simulink model "One_level_boost_igbt_shortcircuit"  (R2022a)
settings: Solver=VariableStepAuto  StartTime=0.0  StopTime=10  MaxStep=10e-6  RelTol=1e-3
libraries: spsSeriesRLCBranchLib x3, spsCurrentMeasurementLib x2, spsDiodeLib x1, spsIdealSwitchLib x1, spsDCVoltageSourceLib x1, spsVoltageMeasurementLib x1, spspowerguiLib x1
settings Model: Creator=Andris  LastModifiedBy=Andris

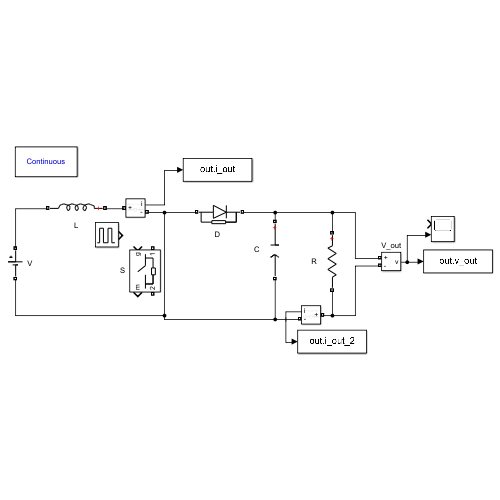
[thumbnail: Simulink's stored preview of the top-level diagram]
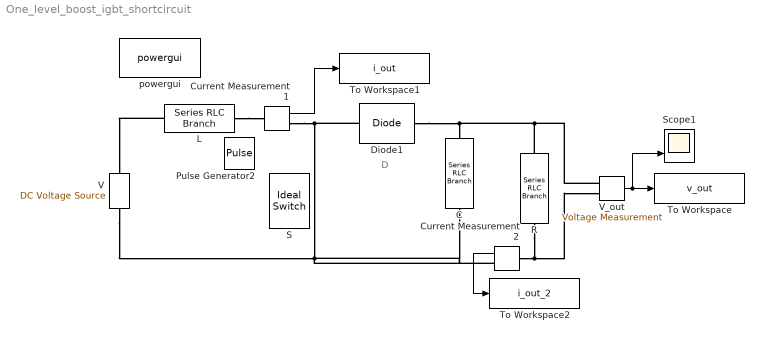
== system One_level_boost_igbt_shortcircuit ==
  note: D
  C : spsSeriesRLCBranchLib/Series RLC Branch  LConnTagsString=__new0  RConnTagsString=__new0  BranchType=C  Resistance=1  Inductance=1e-3  SetiL0=off  InitialCurrent=0  Capacitance=220e-6  Setx0=off  InitialVoltage=Vop1  Measurements=None
  Current Measurement1 : spsCurrentMeasurementLib/Current Measurement  PhasorSimulation=off  OutputType=Complex  PSBequivalent=0
  Current Measurement2 : spsCurrentMeasurementLib/Current Measurement  PhasorSimulation=off  OutputType=Complex  PSBequivalent=0
  Diode1 : spsDiodeLib/Diode  Ron=0  Lon=0  Vf=0  IC=0  UseSnubber=off  Rs=100000  Cs=inf  Measurements=off
  L : spsSeriesRLCBranchLib/Series RLC Branch  LConnTagsString=__new0  RConnTagsString=__new0  BranchType=L  Resistance=1  Inductance=50e-6  SetiL0=off  InitialCurrent=0  Capacitance=1e-6  Setx0=off  InitialVoltage=0  Measurements=None
  Pulse Generator2 : DiscretePulseGenerator  PulseType=Time based  Period=1/48000  PulseWidth=50
  R : spsSeriesRLCBranchLib/Series RLC Branch  LConnTagsString=__new0  RConnTagsString=__new0  BranchType=R  Resistance=12.5  Inductance=1e-3  SetiL0=off  InitialCurrent=0  Capacitance=1e-6  Setx0=off  InitialVoltage=0  Measurements=None
  S : spsIdealSwitchLib/Ideal Switch  Ron=0.001  Lon=0  IC=0  Rs=1e5  Cs=inf  Measurements=on
  Scope1 : Scope  NumInputPorts=2
  To Workspace : ToWorkspace  VariableName=v_out  SampleTime=0.0005
      settings: MaxDataPoints=18000  Save2DSignal=2-D array (concatenate along first dimension)
  To Workspace1 : ToWorkspace  VariableName=i_out  SampleTime=0.0005
      settings: MaxDataPoints=18000  Save2DSignal=2-D array (concatenate along first dimension)
  To Workspace2 : ToWorkspace  VariableName=i_out_2  SampleTime=0.0005
      settings: MaxDataPoints=18000  Save2DSignal=2-D array (concatenate along first dimension)
  V : spsDCVoltageSourceLib/DC Voltage Source  Amplitude=5  Measurements=None
  V_out : spsVoltageMeasurementLib/Voltage Measurement  PhasorSimulation=off  OutputType=Complex  PSBequivalent=0
  powergui : spspowerguiLib/powergui  Priority=1  SimulationMode=Continuous  SampleTime=50e-6  frequency=60  Iterations=50  frequencyindice=0  Pbase=100e6  ErrMax=1e-4  UnitsV=kV  UnitsW=MW  buscounter=0  FunctionMessages=off  echomessages=off  EnableUseOfTLC=off  CurrentSourceSwitches=off  DisableSnubberDevices=off  DisableRonSwitches=off  DisableVfSwitches=off  DisplayEquations=off  AutomaticDiscreteSolvers=off  SolverType=Tustin/Backward Euler (TBE)  Interpol=off  ExternalGateDelay=off  methode=off  Ts=100  x0status=blocks  SPID=on  SwTol=0  HookPort=off  NonlinearTolerance=1e-4  nMaxIteration=100  ContinueOnMaxIteration=off  RestoreLinks=warning  ResistiveCurrentMeasurement=off  Frange=[0:2:500]  Ylog=off  Xlog=on  ShowGrid=off  save=off  variable=ZData  structure=0  ZoomFFT=off  StartTime=0.0  cycles=1  DisplayStyle=1  fundamental=60  FreqAxis=off  MaxFrequency=1000  frequencyindicesteady=1  RmsSteady=1  display=off
  wires:
  V_out/1 -> Scope1/2, To Workspace/1
  Current Measurement1/1 -> To Workspace1/1
  Current Measurement2/1 -> To Workspace2/1
  connections:
  L/RConn1 -- V/RConn1
  L/LConn1 -- Current Measurement1/LConn1
  V_out/LConn1 -- Diode1/RConn1 -- C/LConn1 -- R/LConn1
  Current Measurement1/RConn1 -- V/LConn1 -- C/RConn1 -- Current Measurement2/RConn1 -- Diode1/LConn1
  Current Measurement2/LConn1 -- R/RConn1 -- V_out/LConn2
